simulink model "t2"  (R2024b)
settings: Solver=VariableStepAuto  StartTime=0.0  StopTime=35  RelTol=1e-3
libraries: simulink x1
settings Model: Creator=juanj  LastModifiedBy=juanj

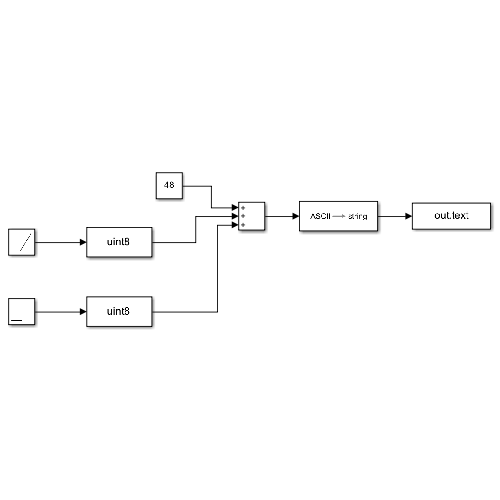
[thumbnail: Simulink's stored preview of the top-level diagram]
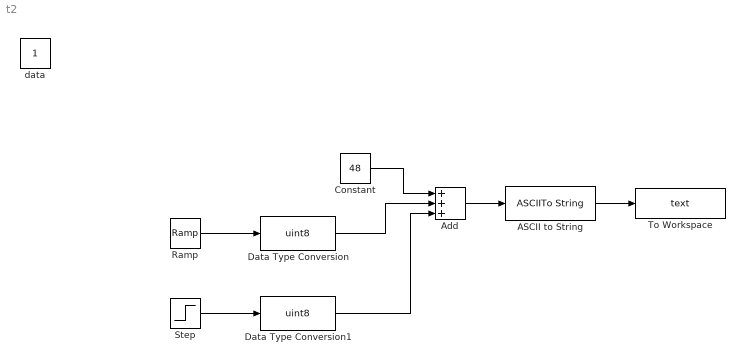
== system t2 ==
  ASCII to String : ASCIIToString
  Add : Sum  Inputs=+++
  Constant : Constant  Value=48  OutDataTypeStr=uint8
  Data Type Conversion : DataTypeConversion  OutDataTypeStr=uint8  SaturateOnIntegerOverflow=off  RndMeth=Floor
  Data Type Conversion1 : DataTypeConversion  OutDataTypeStr=uint8  SaturateOnIntegerOverflow=off  RndMeth=Floor
  Ramp : simulink/Sources/Ramp  slope=1  start=0  InitialOutput=0
  Step : Step  Time=10  After=7  SampleTime=0
  To Workspace : ToWorkspace  VariableName=text  SampleTime=1
  data : Constant  IOType=siggen
  wires:
  ASCII to String/1 -> To Workspace/1
  Constant/1 -> Add/1
  Add/1 -> ASCII to String/1
  Ramp/1 -> Data Type Conversion/1
  Data Type Conversion/1 -> Add/2
  Step/1 -> Data Type Conversion1/1
  Data Type Conversion1/1 -> Add/3
